simulink library "snellDotPosition_ul"  (R2018b)
settings: Solver=VariableStepAuto  StartTime=0.0  StopTime=10.0  RelTol=1e-3
values from neighbouring files (symbols this model uses):
  cameraFOV_rad = cameraFOV_deg*pi/180    [snellDotPosition_init.m]    (also in snellDotPosition_ts.m = [40 20]*pi/180)
  grnd2CamRotMat = calculateRotationMatrix(roll,pitch,yaw)    [rayTrace_ts.m]    (also in rayTrace_ts1.m; rayTrace_ts2.m; snellDotPosition_init.m = calculateRotationMatrix(     cameraEulerAngles_rad(1),     c; snellDotPosition_ts.m)
settings Model: Creator=mcobb  LastModifiedBy=MAE-NCSUCORE

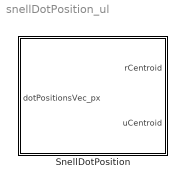
== system snellDotPosition_ul ==
  SnellDotPosition : Subsystem  mask{camPosVec_cm=[-17 0 -5], cameraEulerAngles_deg=[0 135 180], cameraFOV_deg=[40 20], imageDims_px=[1000 2000], dist2Glass=5, indOfRef=[1.000293,1.52,1.333], glassPlane=xy, glassThickness=2}
      mask prompts: camPosVec_cm "Camera Position Vector"; cameraEulerAngles_deg "Camera Euler Angles, deg [roll pitch yaw]"; cameraFOV_deg "Camera Field of View Angle Vec, deg [horiz vert]"; imageDims_px "Image Dimensions, px [rows cols]"; dist2Glass "Distance From Camera To Glass"; indOfRef "Indices of refraction [air glass water]"; glassPlane "Glass Plane"; glassThickness "Glass Thickness, cm"
      mask init:
      | snellDotPosition_init
      mask TypeOptions glassPlane: xy | xz

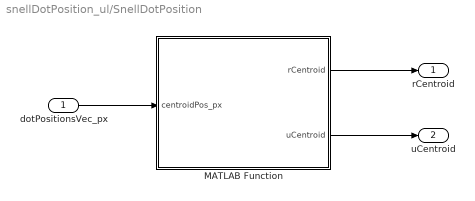
== system snellDotPosition_ul/SnellDotPosition ==
  dotPositionsVec_px : Inport
  MATLAB Function : MATLAB Function  TreatAsAtomicUnit=on
  rCentroid : Outport
  uCentroid : Outport  Port=2
  wires:
  dotPositionsVec_px/1 -> MATLAB Function/1(centroidPos_px)
  MATLAB Function/1(rCentroid) -> rCentroid/1
  MATLAB Function/2(uCentroid) -> uCentroid/1

== matlab function snellDotPosition_ul/SnellDotPosition/MATLAB Function ==
  data: centroidPos_px input; rCentroid output; camPosVec_cm parameter; grnd2CamRotMat parameter; cameraFOV_rad parameter; imageDims_px parameter; dist2Glass parameter; indOfRef parameter; glassPlane parameter; glassThickness parameter; uCentroid output
function [rCentroid,uCentroid] = ...
    snellDotPosition(...
    centroidPos_px,camPosVec_cm,grnd2CamRotMat,cameraFOV_rad,...
    imageDims_px,dist2Glass,indOfRef,glassPlane,glassThickness)

[rCentroid,uCentroid] = ...
    snellDotPosition(...
    centroidPos_px,camPosVec_cm,grnd2CamRotMat,cameraFOV_rad,...
    imageDims_px,dist2Glass,indOfRef,glassPlane,glassThickness);

end
